simulink model "second_order_testing_simulation"  (R2023a)
settings: Solver=VariableStepAuto  StartTime=0.0  StopTime=10.0  MaxStep=1e-6
settings Model: Creator=mazen  LastModifiedBy=mazen

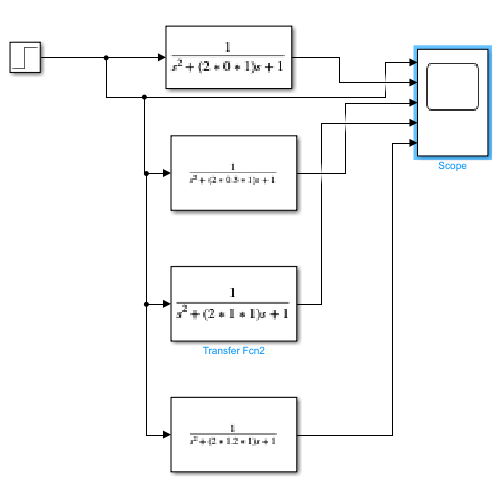
[thumbnail: Simulink's stored preview of the top-level diagram]
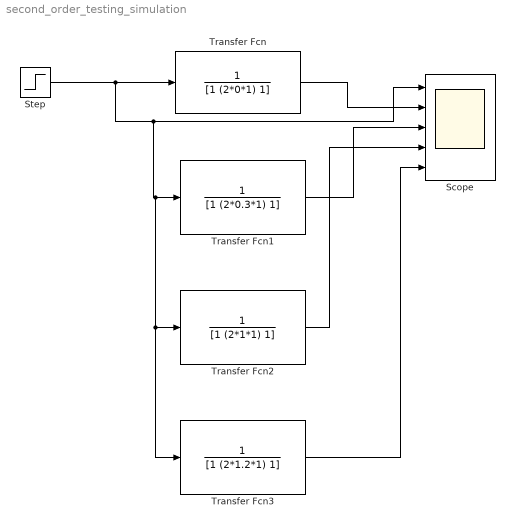
== system second_order_testing_simulation ==
  Scope : Scope  NumInputPorts=5
  Step : Step  SampleTime=0
  Transfer Fcn : TransferFcn  Denominator=[1 (2*0*1) 1]
  Transfer Fcn1 : TransferFcn  Denominator=[1 (2*0.3*1) 1]
  Transfer Fcn2 : TransferFcn  Denominator=[1 (2*1*1) 1]
  Transfer Fcn3 : TransferFcn  Denominator=[1 (2*1.2*1) 1]
  wires:
  Step/1 -> Transfer Fcn3/1, Transfer Fcn2/1, Transfer Fcn1/1, Scope/1, Transfer Fcn/1
  Transfer Fcn/1 -> Scope/2
  Transfer Fcn1/1 -> Scope/3
  Transfer Fcn2/1 -> Scope/4
  Transfer Fcn3/1 -> Scope/5
